simulink model "OW1_2G_HIL"  (R2025b)
settings: Solver=ode4  StartTime=0  StopTime=240  FixedStep=0.0001  MaxStep=0.0001  RelTol=1e-3
values from neighbouring files (symbols this model uses):
  simu = simulationClass()    [wecSimInputFile.m]
  waves = waveClass("noWaveCIC")    [wecSimInputFile.m]
  wecSimModelRate = 0.002    [wecSimInputFile.m]
undefined symbols (not defined in the file or in its folder): body, cable, constraint, geometry, hydroData, pto, X, Y, Z
libraries: sm_lib x8, slrealtimeloglib x2, WECSim_Lib_Cables x2, nesl_utility x2, custom_WECSim_Lib_Body_Elements_612 x2, WECSim_Lib_Constraints x2, SG_DLE_position_control_module_hose_pump x1, dspstat3 x1
settings Model: Creator=cmmcguir  LastModifiedBy=cmmcguir
settings SolverCC: ConcurrentTasks=on  ZeroCrossControl=DisableAll  PositivePriorityOrder=on  AutoInsertRateTranBlk=on
settings DataIOCC: InspectSignalLogs=on  ReturnWorkspaceOutputs=off
settings OptimizationCC: BlockReduction=off  OptimizeBlockIOStorage=off  SimCompilerOptimization=on
settings DebuggingCC: TasksWithSamePriorityMsg=none
settings HardwareCC: ProdBitPerLong=64.0  ProdLongLongMode=on  ProdHWDeviceType=Intel->x86-64 (Linux 64)
settings RTWCC: SystemTargetFile=speedgoat.tlc  TemplateMakefile=slrealtime_default_tmf  Toolchain=Simulink Real-Time Toolchain  BuildConfiguration=Faster Runs  CodeExecutionProfiling=on  TargetLang=C++  GPUComputeCapability=3.5  Description=Speedgoat Real-Time Target Machine
settings SimulinkRealTimeTargetCC: SLRTFileLogMaxRuns=1.0  ExtModeMaxTrigDuration=10.0  ExtModeStaticAllocSize=1000000.0  ExtModeTransport=0.0  MultiwordLength=2048.0  DynamicStringBufferSize=256.0  PreserveMATLABNamespacesInGeneratedCode=on  SubcomponentCodeInterfacePackaging=Reusable function  MATLABClassNameForMDSCustomization=Simulink.SoftwareTarget.GRTCustomization  InstructionSetFMA=off  LogToMDFFile=off
settings SimscapeCC: SimscapeLogLimitData=off
settings ExplorerConfigSet: SimMechanicsOpenEditorOnUpdate=off

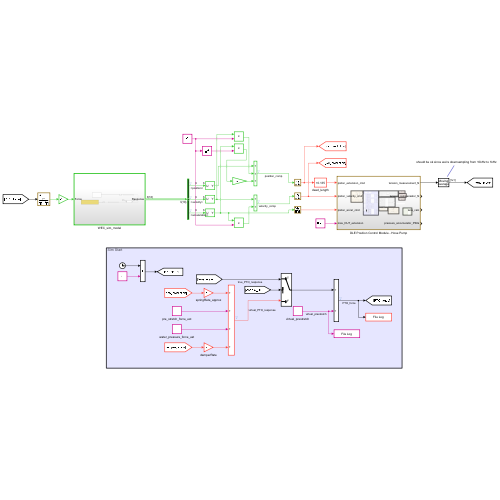
[thumbnail: Simulink's stored preview of the top-level diagram]
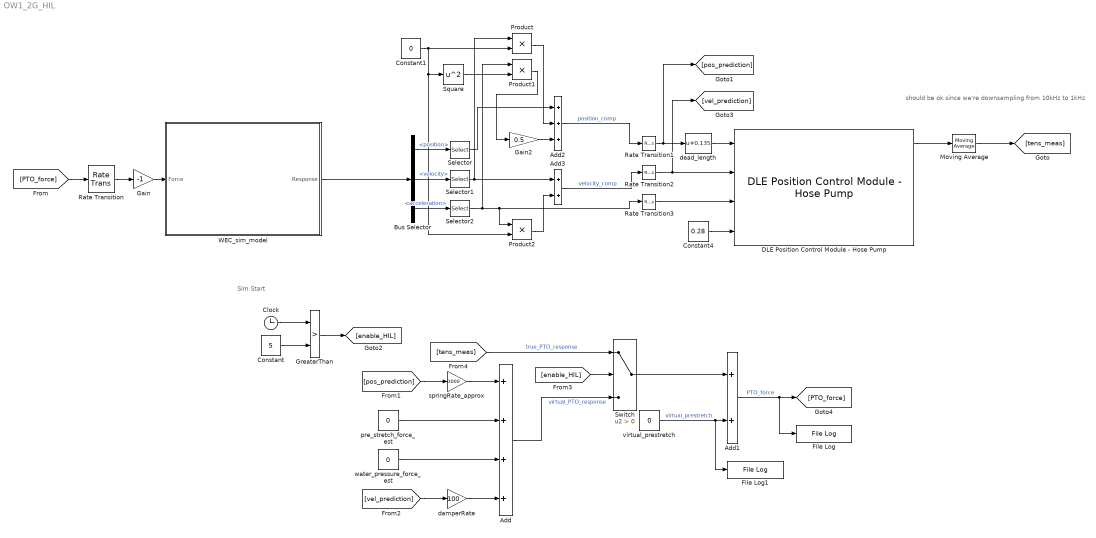
== system OW1_2G_HIL ==
  note: should be ok since we're downsampling from 10kHz to 1kHz
  note: Sim Start
  Add : Sum  Inputs=++++
  Add1 : Sum
  Add2 : Sum  Inputs=+++
  Add3 : Sum
  Bus Selector : BusSelector  OutputSignals=position,velocity,acceleration
  Clock : Clock
  Constant : Constant  Value=5
  Constant1 : Constant  Value=0
  Constant4 : Constant  Value=0.28
  DLE Position Control Module - Hose Pump : SG_DLE_position_control_module_hose_pump/DLE Position Control Module - Hose Pump  SystemSampleTime=-1  VariantActivationTime=update diagram  EmptyChoice=off  PassThrough=off  PassThroughVariantControl=(default)  EmptyChoiceVariantControl=(default)  AllowFlexibleInterface=on  Latency=0  AutoFrameSizeCalculation=off
      link override "Analog input ": parAdcRanges=[3 3 3 3 3 3 3 3]
  File Log : slrealtimeloglib/File Log  decimation=1  inputProcessing=Elements as channels (sample based)
  File Log1 : slrealtimeloglib/File Log  decimation=1  inputProcessing=Elements as channels (sample based)
  Gain : Gain  Gain=-1
  Gain2 : Gain  Gain=0.5
  GreaterThan : RelationalOperator  Operator=>  OutDataTypeStr=boolean  RndMeth=Simplest  InputSameDT=off
  Moving Average : dspstat3/Moving Average  Method=Sliding window  ForgettingFactorPort=off  SpecifyWindowLength=on  WindowLength=10  OverlapLength=9  AllowArbitraryInputLength=off  ForgettingFactor=0.9  SimulateUsing=Interpreted execution
  Product : Product
  Product1 : Product
  Product2 : Product
  Rate Transition : RateTransition  OutPortSampleTime=wecSimModelRate
  Rate Transition1 : RateTransition  OutPortSampleTime=simu.dt
  Rate Transition2 : RateTransition  OutPortSampleTime=simu.dt
  Rate Transition3 : RateTransition  OutPortSampleTime=simu.dt
  Selector : Selector  InputPortWidth=6  IndexOptions=Index vector (dialog)  Indices=3  OutputSizes=1
  Selector1 : Selector  InputPortWidth=6  IndexOptions=Index vector (dialog)  Indices=3  OutputSizes=1
  Selector2 : Selector  InputPortWidth=6  IndexOptions=Index vector (dialog)  Indices=3  OutputSizes=1
  Square : Math  Operator=square
  Switch : Switch  Criteria=u2 > Threshold  SaturateOnIntegerOverflow=off  InputSameDT=off
  WEC_sim_model : Subsystem  TreatAsAtomicUnit=on  SystemSampleTime=wecSimModelRate
  damperRate : Gain  Gain=100
  dead_length : Bias  Bias=0.135  SaturateOnIntegerOverflow=off
  pre_stretch_force_est : Constant  Value=0
  springRate_approx : Gain  Gain=3000
  virtual_prestretch : Constant  Value=0
  water_pressure_force_est : Constant  Value=0
  wires:
  Constant4/1 -> DLE Position Control Module - Hose Pump/4
  Selector/1 -> Add2/1
  Bus Selector/1 -> Selector/1  "<position>"
  Bus Selector/2 -> Selector1/1  "<velocity>"
  Selector2/1 -> Product1/1, Product2/1, Rate Transition3/1
  Bus Selector/3 -> Selector2/1  "<acceleration>"
  Rate Transition/1 -> Gain/1
  WEC_sim_model/1(Response) -> Bus Selector/1
  Gain/1 -> WEC_sim_model/1(Force)
  dead_length/1 -> DLE Position Control Module - Hose Pump/1
  Rate Transition1/1 -> dead_length/1, [pos_prediction]
  Rate Transition2/1 -> [vel_prediction], DLE Position Control Module - Hose Pump/2
  Rate Transition3/1 -> DLE Position Control Module - Hose Pump/3
  Moving Average/1 -> [tens_meas]
  [enable_HIL] -> Switch/2
  [pos_prediction] -> springRate_approx/1
  Add/1 -> Switch/3  "virtual_PTO_response"
  Constant/1 -> GreaterThan/2
  pre_stretch_force_est/1 -> Add/2
  GreaterThan/1 -> [enable_HIL]
  Clock/1 -> GreaterThan/1
  Add1/1 -> File Log/1, [PTO_force]  "PTO_force"
  Switch/1 -> Add1/1
  damperRate/1 -> Add/4
  [tens_meas] -> Switch/1  "true_PTO_response"
  springRate_approx/1 -> Add/1
  [vel_prediction] -> damperRate/1
  virtual_prestretch/1 -> File Log1/1, Add1/2  "virtual_prestretch"
  water_pressure_force_est/1 -> Add/3
  [PTO_force] -> Rate Transition/1
  DLE Position Control Module - Hose Pump/1 -> Moving Average/1
  Add2/1 -> Rate Transition1/1  "position_comp"
  Selector1/1 -> Add3/1, Product/1
  Gain2/1 -> Add2/3
  Add3/1 -> Rate Transition2/1  "velocity_comp"
  Constant1/1 -> Product2/2, Square/1, Product/2
  Product/1 -> Add2/2
  Square/1 -> Product1/2
  Product1/1 -> Gain2/1
  Product2/1 -> Add3/2

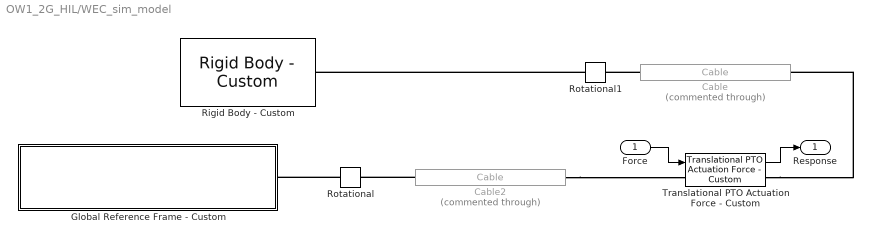
== system OW1_2G_HIL/WEC_sim_model ==
  Force : Inport
  Cable : WECSim_Lib_Cables/Cable  Commented=through  VariantControl=sv_Cable3DOF  cable=cable(1)  baseConnectionName=constraint(1)  followerConnectionName=constraint(2)  stiffness=0  damping=0  length=0  preTension=0  diplacement=0 0 0  axis=0 1 0  angle=0  y=0 1 0  z=0 0 1
      settings: AttributesFormatString=%<cable>
  Cable2 : WECSim_Lib_Cables/Cable  Commented=through  VariantControl=sv_Cable3DOF  cable=cable(2)  baseConnectionName=constraint(1)  followerConnectionName=constraint(2)  stiffness=0  damping=0  length=0  preTension=0  diplacement=0 0 0  axis=0 1 0  angle=0  y=0 1 0  z=0 0 1
      settings: AttributesFormatString=%<cable>
  Global Reference Frame - Custom : Subsystem  mask(Frames){waves=waves, simu=simu, InputMethod=Input File, InputFile=wecSimInputFile.m, mode=normal, explorer=off, solver=ode4, startTime=0, rampTime=100, endTime=400, dt=0.1, cicEndTime=60, stateSpace=0, WaveClass=regular, height=2.5, period=8, elevationFile=NOT DEFINED, spectrumFile=NOT DEFINED, direction=0, spread=1, spectrumType=NOT DEFINED, phaseSeed=0, option=EqualEnergy}
      mask prompts: waves "Wave Class Name"; simu "Simulation Class Name"; InputMethod "Parameter Input Method"; mode "Simulation Mode:"; explorer "SimMechanics Explorer:"; solver "SimSolver:"; startTime "Start Time [s]:"; rampTime "Ramp Time [s]:"; endTime "End Time [s]:"; dt "Step Size [s]:"; cicEndTime "CI Time [s]:"; stateSpace "Turn on State Space"; WaveClass "Select Wave Class:"; height "Wave Height [m]:"; period "Wave Period [s]:"; direction "Wave Direction [deg]:"; spread "Wave Spread [0-1]:"; spectrumType "Wave Spectrum Type:"; phaseSeed "Phase Seed:"; option "Frequency Discretization:"
      mask help:
      | This block contains Global References, including solver configurations, free surface and seabed description, and simulation time.
      | It uses the following fields from the Simulation and Wave classes:
      |
      | Simulation Class:
      |     .endTime
      |     .dt
      |     .domainSize
      |
      | Wave Class:
      |     .waterDepth
      mask Help:
      | This block contains Global References, including solver configurations, free surface and seabed description, and simulation time.
      | It uses the following fields from the Simulation and Wave classes:
      | 
      | Simulation Class:
      |     .endTime
      |     .dt
      |     .domainSize
      | 
      | Wave Class:
      |     .waterDepth
      mask TypeOptions InputMethod: Input File | Custom Parameters
      mask Callback InputMethod: inputOrCustomCallback(gcbh)
      mask TypeOptions mode: normal | accelerator | rapid-accelerator
      mask TypeOptions explorer: on | off
      mask TypeOptions solver: ode4 | ode45
      mask TypeOptions stateSpace: 0 | 1
      mask TypeOptions WaveClass: noWaveCIC | regular | regularCIC | irregular | spectrumImport | etaImport
      mask Callback WaveClass: waveClassCallback(gcbh)
      mask TypeOptions spectrumType: PM | JS | NOT DEFINED
      mask TypeOptions option: EqualEnergy | Traditional
      mask DialogControl InputFileGroup Prompt: Input File
      mask DialogControl InFileButton Prompt: Select File
      mask DialogControl InFileButton Callback: inFileButtonCallback(gcbh)
      mask DialogControl CustomParameterGroup Prompt: Custom Parameters
      mask DialogControl LoadParam Prompt: Load parameters from Input File
      mask DialogControl LoadParam Callback: loadInputFileCallback(gcbh)
      mask DialogControl SimData Prompt: Simulation Data
      mask DialogControl WaveInfo Prompt: Wave Information
      mask DialogControl ETAbutton Prompt: Select etaData.mat file
      mask DialogControl ETAbutton Callback: etaButtonCallback(gcbh)
      mask DialogControl SpecButton Prompt: Select spectrumData.mat file
      mask DialogControl SpecButton Callback: spectrumButtonCallback(gcbh)
      mask Display: fprintf('Active Method: \n%s',get_param(gcbh,'InputMethod'))
  Rigid Body - Custom : custom_WECSim_Lib_Body_Elements_612/Rigid Body - Custom  body=body(1)  h5File=hydroData/*.h5  geometryFile=geometry/*.stl  mass=0  inertia=0 0 0  inertiaProducts=0 0 0  nonHydro=0  nonlinearHydro=0  centerGravity=0 0 0  centerBuoyancy=0 0 0  dof=6  volume=0  QTFs=0  displacement=0 0 0  axis=0 1 0  angle=0  option=0  cd=0 0 0  ca=0 0 0  area=0 0 0  VME=0  rgME=0 0 0  z=0 0 1
      settings: AttributesFormatString=%<body>
  Rotational : WECSim_Lib_Constraints/Rotational  constraint=constraint(1)  loc="0  0  0"  displacement=0 0 0  y=0 1 0  z=0 0 1  upperLimitSpecify=off  upperLimitBound=0  upperLimitTransitionRegionWidth=0  upperLimitStiffness=0  upperLimitDamping=0  lowerLimitSpecify=off  lowerLimitBound=0  lowerLimitTransitionRegionWidth=0  lowerLimitStiffness=0  lowerLimitDamping=0
      settings: AttributesFormatString=%<constraint>
  Rotational1 : WECSim_Lib_Constraints/Rotational  constraint=constraint(2)  loc="0  0  0"  displacement=0 0 0  y=0 1 0  z=0 0 1  upperLimitSpecify=off  upperLimitBound=0  upperLimitTransitionRegionWidth=0  upperLimitStiffness=0  upperLimitDamping=0  lowerLimitSpecify=off  lowerLimitBound=0  lowerLimitTransitionRegionWidth=0  lowerLimitStiffness=0  lowerLimitDamping=0
      settings: AttributesFormatString=%<constraint>
  Translational PTO Actuation Force - Custom : custom_WECSim_Lib_Body_Elements_612/Translational PTO Actuation Force - Custom  pto=pto(1)  loc="0  0  0"  stiffness=0  damping=0  equilibriumPosition=0  pretension=0  displacement=0 0 0  y=0 1 0  z=0 0 1  upperLimitSpecify=off  upperLimitBound=0  upperLimitTransitionRegionWidth=0  upperLimitStiffness=0  upperLimitDamping=0  lowerLimitSpecify=off  lowerLimitBound=0  lowerLimitTransitionRegionWidth=0  lowerLimitStiffness=0  lowerLimitDamping=0
      settings: AttributesFormatString=%<pto>
  Response : Outport
  wires:
  Translational PTO Actuation Force - Custom/1 -> Response/1
  Force/1 -> Translational PTO Actuation Force - Custom/1
  connections:
  Rotational1/RConn1 -- Rigid Body - Custom/RConn1
  Cable/RConn1 -- Rotational1/LConn1
  Rotational/LConn1 -- Global Reference Frame - Custom/RConn1
  Translational PTO Actuation Force - Custom/RConn1 -- Cable/LConn1
  Cable2/RConn1 -- Translational PTO Actuation Force - Custom/LConn1
  Cable2/LConn1 -- Rotational/RConn1

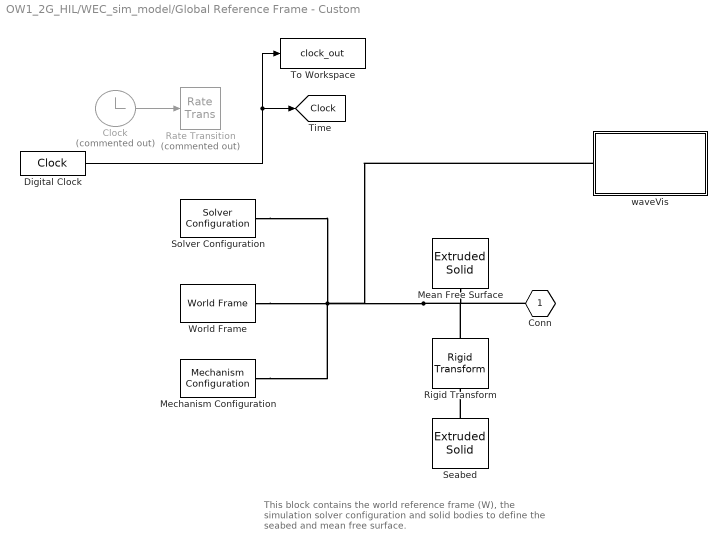
== system OW1_2G_HIL/WEC_sim_model/Global Reference Frame - Custom ==
  note: This block contains the world reference frame (W), the simulation solver configuration and
      | solid bodies to define the seabed and mean free surface.
  Clock : Clock  Commented=on
  Digital Clock : DigitalClock  SampleTime=wecSimModelRate
  Mean Free Surface : sm_lib/Body Elements/Extruded Solid  ExtrusionType=General  PolygonNumSides=3  PolygonOuterRadius=1  PolygonOuterRadiusUnits=m  ExportEntireGeometry=off  ExtrusionCrossSection=[simu.domainSize simu.domainSize; -simu.domainSize simu.domainSize; -simu.domainSize -simu.domainSize; simu.domainSize -simu.domainSize]  ExtrusionCrossSectionUnits=m  ExportConvexHullGeometry=off  ExtrusionLength=simu.domainSize/200  ExtrusionLengthUnits=m  InertiaType=Custom  BasedOnType=Density  Density=1000  DensityUnits=kg/(m^3)  Mass=10^20  MassUnits=kg  CenterOfMass=[0 0 0]  CenterOfMassUnits=m  MomentsOfInertia=[10^20 10^20 10^20]  MomentsOfInertiaUnits=kg*m^2  ProductsOfInertia=[0 0 0]  ProductsOfInertiaUnits=kg*m^2  GraphicType=FromGeometry  MarkerShape=Sphere  MarkerSize=10  GraphicVisPropType=SimpleVisualProperties  GraphicDiffuseColor=[0.0 0.6 0.8]  GraphicOpacity=0.3  GraphicSpecularColor=[0.5 0.5 0.5 1.0]  GraphicAmbientColor=[0.15 0.15 0.15 1.0]  GraphicEmissiveColor=[0.0 0.0 0.0 1.0]  GraphicShininess=75  DoExposeReferenceFrame=on  SerializedFrames=<Frames/>
  Mechanism Configuration : sm_lib/Utilities/Mechanism Configuration  UniformGravity=Constant  GravityVector=[0 0 0]  GravityVectorUnits=m/s^2  LinearizationDelta=0.001  JointModeTransitionNonlinearIterations=2
  Rate Transition : RateTransition  Commented=on  OutPortSampleTime=wecSimModelRate
  Rigid Transform : sm_lib/Frames and Transforms/Rigid Transform  RotationMethod=None  FollAlignAxisA=+X  BaseAlignAxisA=+Y  FollAlignAxisB=+Y  BaseAlignAxisB=+Z  RotationStandardAxis=+Z  RotationAngle=0  RotationAngleUnits=deg  RotationArbitraryAxis=[0 0 1]  RotationSequenceAxes=FollowerAxes  RotationSequence=XYX  RotationSequenceAngles=[0 0 0]  RotationSequenceAnglesUnits=deg  RotationMatrix=[1 0 0; 0 1 0; 0 0 1]  Quaternion=[1 0 0 0]  TranslationMethod=Cartesian  TranslationCartesianOffset=[0 0 -waves(1).waterDepth]  TranslationCartesianOffsetUnits=m  TranslationStandardAxis=+Z  TranslationStandardOffset=0  TranslationStandardOffsetUnits=m  TranslationROffset=0  TranslationROffsetUnits=m  TranslationThetaOffset=0  TranslationThetaOffsetUnits=deg  TranslationZOffset=0  TranslationZOffsetUnits=m
  Seabed : sm_lib/Body Elements/Extruded Solid  ExtrusionType=General  PolygonNumSides=3  PolygonOuterRadius=1  PolygonOuterRadiusUnits=m  ExportEntireGeometry=off  ExtrusionCrossSection=[simu.domainSize simu.domainSize; -simu.domainSize simu.domainSize; -simu.domainSize -simu.domainSize; simu.domainSize -simu.domainSize]  ExtrusionCrossSectionUnits=m  ExportConvexHullGeometry=off  ExtrusionLength=simu.domainSize/100  ExtrusionLengthUnits=m  InertiaType=Custom  BasedOnType=Density  Density=1000  DensityUnits=kg/(m^3)  Mass=10^20  MassUnits=kg  CenterOfMass=[0 0 0]  CenterOfMassUnits=m  MomentsOfInertia=[10^20 10^20 10^20]  MomentsOfInertiaUnits=kg*m^2  ProductsOfInertia=[0 0 0]  ProductsOfInertiaUnits=kg*m^2  GraphicType=FromGeometry  MarkerShape=Sphere  MarkerSize=10  GraphicVisPropType=SimpleVisualProperties  GraphicDiffuseColor=[0.4 0.4 0.0]  GraphicOpacity=1  GraphicSpecularColor=[0.5 0.5 0.5 1.0]  GraphicAmbientColor=[0.15 0.15 0.15 1.0]  GraphicEmissiveColor=[0.0 0.0 0.0 1.0]  GraphicShininess=75  DoExposeReferenceFrame=on  SerializedFrames=<Frames/>
  Solver Configuration : nesl_utility/Solver Configuration  PhysicalDomain=network_engine_domain  SubClassName=solver  LeftPortType=input  RightPortType=generic  Tones=[]  Harmonics=[]  SimulateNoise=off  Profile=off  UseLocalSampling=off  EnableSwitchedLinearOptims=on  FrequencyDomain=off  UseCCode=off  RelTol=0.001  AbsTol=1e-06  MinStep=1e-09  ToWorkspace=off  RevertToSquareIcSolve=off  NumHomotopyIterations=100  PhasorMode=off  PhasorModeNumHarmonics=1  ConsistencySolver=NEWTON_FTOL  IndexReductionMethod=DerivativeReplacement  DoDC=on  ResidualTolerance=1e-9  ConsistencyTolSource=GLOBAL  ConsistencyAbsTol=0.001  ConsistencyRelTol=0.001  ConsistencyTolFactor=0.001  UseLocalSolver=on  LocalSolverChoice=NE_BACKWARD_EULER_ADVANCER  ResolveIndetEquations=on  FunctionEvalNumThread=1  LocalSolverSampleTime=wecSimModelRate  DoFixedCost=off  MaxNonlinIter=3  MaxModeIter=2  ComputeImpulses=off  ImpulseIterations=2  LinearAlgebra=Sparse  LinearAlgebraNumThread=0  EquationFormulation=NE_TIME_EF  DelaysMemoryBudget=1024  AutomaticFiltering=on  FilteringTimeConstant=0.001  PartitionStorageMethod=AS_NEEDED  PartitionMemoryBudget=1024  PartitionMethod=FAST  MultibodyUseLocalSolver=on  MultibodyLocalSolverChoice=ODE4  MultibodyLocalSolverSampleTime=wecSimModelRate
  To Workspace : ToWorkspace  VariableName=clock_out  SaveFormat=Structure With Time  SampleTime=-1
  World Frame : sm_lib/Frames and Transforms/World Frame
  waveVis : Subsystem  Variant=on  VariantControl=Choice  EmptyChoice=on  PropagateVariantConditions=on
  Conn : PMIOPort  Side=Right
  tag scope: Clock=global
  wires:
  Clock/1 -> Rate Transition/1
  Digital Clock/1 -> To Workspace/1, [Clock]
  connections:
  World Frame/RConn1 -- Mechanism Configuration/RConn1 -- waveVis/LConn1 -- Conn/RConn1 -- Mean Free Surface/RConn1 -- Rigid Transform/LConn1 -- Solver Configuration/RConn1
  Seabed/RConn1 -- Rigid Transform/RConn1

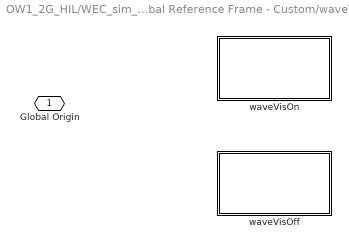
== system OW1_2G_HIL/WEC_sim_model/Global Reference Frame - Custom/waveVis ==
  waveVisOff : Subsystem  VariantControl=sv_visualizationOFF
  waveVisOn : Subsystem  VariantControl=sv_visualizationON
  Global Origin : PMIOPort  Side=Left

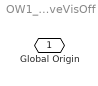
== system OW1_2G_HIL/WEC_sim_model/Global Reference Frame - Custom/waveVis/waveVisOff ==
  Global Origin : PMIOPort  Side=Left

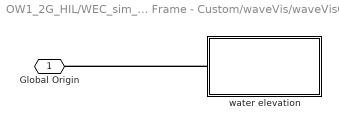
== system OW1_2G_HIL/WEC_sim_model/Global Reference Frame - Custom/waveVis/waveVisOn ==
  water elevation : Subsystem  mask{waves=waves}
      mask prompts: waves "Waves Object"
      mask init:
      | cb = gcb;
      | nWaves = length(waves);
      | 
      | for i = 1:nWaves
      |     loc = waves(i).marker.location;
      |     nGauges = size(loc,1);
      |     for iWG = 1:nGauges
      |         try 
      |             find_system([cb,'/marker_', num2str(i), num2str(iWG)],'Type','Block');
      |         catch
      |             add_block  ([cb,'/marker1'],[cb,'/marker_', num2str(i), num2str(iWG)],'MakeNameUnique','off',...
      |                        'Position',[0,100*iWG + iWG*3, 180 + iWG*3, 40+100*iWG + iWG*3],'BackgroundColor','white');
      |     
      |             set_param([cb,'/marker_', num2str(i), num2str(iWG)],'wgT',           sprintf('[waves(%d).waveAmpTimeViz(:,1),waves(%d).waveAmpTimeViz(:,%d)]',i,i,iWG+1));
      |     
      |             set_param([cb,'/marker_', num2str(i), num2str(iWG)],'wgloc',         sprintf('waves(%d).marker.location(%d,:)',i,iWG));
      |             
      |             set_param([cb,'/marker_', num2str(i), num2str(iWG)],'markStyle',      sprintf('waves(%d).marker.style',i));
      |     
      |             set_param([cb,'/marker_', num2str(i), num2str(iWG)],'markSize',       sprintf('waves(%d).marker.size',i));
      |     
      |             set_param([cb,'/marker_', num2str(i), num2str(iWG)],'graphicColor',   sprintf('waves(%d).marker.graphicColor',i));
      |     
      |             add_line(cb,...
      |                 ['marker_', num2str(i), num2str(iWG),'/LConn1'],...
      |                 'Global Origin/RConn1',...
      |                 'autorouting','on');
      |         end
      |     end
      | end
  Global Origin : PMIOPort  Side=Left
  connections:
  water elevation/LConn1 -- Global Origin/RConn1

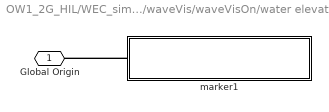
== system OW1_2G_HIL/WEC_sim_model/Global Reference Frame - Custom/waveVis/waveVisOn/water elevation ==
  marker1 : Subsystem  mask{markStyle=waves(1).marker.style, wgloc=waves(1).marker.location(1,:), wgT=[waves(1).waveAmpTimeViz(:,1), waves(1).waveAmpTimeViz(:,2)], markSize=waves(1).marker.size, graphicColor=waves(1).marker.graphicColor}
      mask prompts: markStyle "Marker Style"; wgloc "Wave Gauge Location [X,Y]"; wgT "Wave Gauge Time History"; markSize "Marker Size"; graphicColor "Graphic Color"
  Global Origin : PMIOPort  Side=Left
  connections:
  marker1/LConn1 -- Global Origin/RConn1

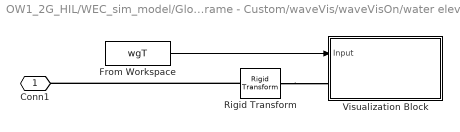
== system OW1_2G_HIL/WEC_sim_model/Global Reference Frame - Custom/waveVis/waveVisOn/water elevation/marker1 ==
  From Workspace : FromWorkspace  VariableName=wgT
  Rigid Transform : sm_lib/Frames and Transforms/Rigid Transform  RotationMethod=None  FollAlignAxisA=+X  BaseAlignAxisA=+Y  FollAlignAxisB=+Y  BaseAlignAxisB=+Z  RotationStandardAxis=+Z  RotationAngle=0.0  RotationAngleUnits=deg  RotationArbitraryAxis=[0 0 1]  RotationSequenceAxes=FollowerAxes  RotationSequence=XYX  RotationSequenceAngles=[0 0 0]  RotationSequenceAnglesUnits=deg  RotationMatrix=[1 0 0; 0 1 0; 0 0 1]  Quaternion=[1 0 0 0]  TranslationMethod=Cartesian  TranslationCartesianOffset=[wgloc 0]  TranslationCartesianOffsetUnits=m  TranslationStandardAxis=+Z  TranslationStandardOffset=0  TranslationStandardOffsetUnits=m  TranslationROffset=0  TranslationROffsetUnits=m  TranslationThetaOffset=0  TranslationThetaOffsetUnits=deg  TranslationZOffset=0  TranslationZOffsetUnits=m
  Visualization Block : Subsystem  mask{markStyle=markStyle, markSize=markSize, graphicColor=graphicColor}
      mask prompts: markStyle "Waves Marker Style"; markSize "Waves Marker Size"; graphicColor "Graphic Color"
      mask init:
      | % Marker Shape %<MarkerShape>
      | % Marker Size %<MarkerSize>%<MarkerSizeUnits>
      | cb = gcb;
      | 
      | set_param([cb '/WaveElevation'],'MarkerSize','markSize')
      | 
      | if markStyle == 1
      |     set_param([cb '/WaveElevation'],'MarkerShape','Sphere')
      | elseif markStyle == 2
      |     set_param([cb '/WaveElevation'],'MarkerShape','Cube')
      | elseif markStyle == 3
      |     set_param([cb '/WaveElevation'],'MarkerShape','Frame')
      | end
      | set_param([cb '/WaveElevation'],'GraphicDiffuseColor','graphicColor')
      | set_param([cb '/WaveElevation'],'GraphicOpacity','.5')
  Conn1 : PMIOPort  Side=Left
  wires:
  From Workspace/1 -> Visualization Block/1(Input)
  connections:
  Rigid Transform/RConn1 -- Visualization Block/LConn1
  Rigid Transform/LConn1 -- Conn1/RConn1

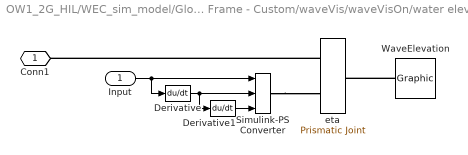
== system OW1_2G_HIL/WEC_sim_model/Global Reference Frame - Custom/waveVis/waveVisOn/water elevation/marker1/Visualization Block ==
  Input : Inport
  Derivative : Derivative
  Derivative1 : Derivative
  Simulink-PS Converter : nesl_utility/Simulink-PS Converter  PhysicalDomain=network_engine_domain  SubClassName=ps_input  LeftPortType=input  RightPortType=output  PseudoPeriodic=off  Frequencies=[]  NoiseDistribution=none  NoiseParameters=[]  Unit=1  AffineConversion=off  FilteringAndDerivatives=provide  SimscapeFilterOrder=1  InputFilterTimeConstant=0.001  UdotUserProvided=2
  WaveElevation : sm_lib/Body Elements/Graphic  GraphicType=Marker  MarkerShape=Sphere  MarkerSize=markSize  GraphicVisPropType=SimpleVisualProperties  GraphicDiffuseColor=graphicColor  GraphicOpacity=.5  GraphicSpecularColor=[0.5 0.5 0.5 1.0]  GraphicAmbientColor=[0.15 0.15 0.15 1.0]  GraphicEmissiveColor=[0.0 0.0 0.0 1.0]  GraphicShininess=75
      settings: AttributesFormatString=|
      | Marker Shape: %<MarkerShape>
      | Marker Size:    %<MarkerSize>%<MarkerSizeUnits>
  eta : sm_lib/Joints/Prismatic Joint  JointMode=Normal  CompositeWrenchDir=FollowerOnBase  CompositeWrenchFrame=BaseFrame  SenseConstraintForce=off  SenseConstraintTorque=off  SenseTotalForce=off  SenseTotalTorque=off  PositionTargetSpecify=off  PositionTargetPriority=High  PositionTargetValue=0  PositionTargetValueUnits=m  VelocityTargetSpecify=off  VelocityTargetPriority=High  VelocityTargetValue=0  VelocityTargetValueUnits=m/s  EquilibriumPosition=0  EquilibriumPositionUnits=m  SpringStiffness=0  SpringStiffnessUnits=N/m  DampingCoefficient=0  DampingCoefficientUnits=N/(m/s)  LowerLimitSpecify=off  LowerLimitBound=-1  LowerLimitBoundUnits=m  LowerLimitStiffness=1e6  LowerLimitStiffnessUnits=N/m  LowerLimitDamping=1e3  LowerLimitDampingUnits=N/(m/s)  LowerLimitTransitionRegionWidth=1e-4  LowerLimitTransitionRegionWidthUnits=m  UpperLimitSpecify=off  UpperLimitBound=1  UpperLimitBoundUnits=m  UpperLimitStiffness=1e6  UpperLimitStiffnessUnits=N/m  UpperLimitDamping=1e3  UpperLimitDampingUnits=N/(m/s)  UpperLimitTransitionRegionWidth=1e-4  UpperLimitTransitionRegionWidthUnits=m  TorqueActuationMode=ComputedTorque  MotionActuationMode=InputMotion  SensePosition=off  SenseVelocity=off  SenseAcceleration=off  SenseTorqueForce=off  SenseLowerLimitTorqueForce=off  SenseUpperLimitTorqueForce=off
  Conn1 : PMIOPort  Side=Left
  wires:
  Input/1 -> Derivative/1, Simulink-PS Converter/1
  Derivative/1 -> Derivative1/1, Simulink-PS Converter/2
  Derivative1/1 -> Simulink-PS Converter/3
  connections:
  Simulink-PS Converter/RConn1 -- eta/LConn2
  WaveElevation/RConn1 -- eta/RConn1
  eta/LConn1 -- Conn1/RConn1
